simulink model "model"  (R2014a)
settings: Solver=VariableStepAuto  StartTime=0.0  StopTime=10.0  RelTol=1e-3
settings Model: Creator=GGX  LastModifiedBy=thinkpad
settings DataIOCC: LimitDataPoints=off  SaveFormat=Dataset
settings OptimizationCC: LifeSpan=auto  SimCompilerOptimization=off
settings DebuggingCC: MergeDetectMultiDrivingBlocksExec=error  SolverPrmCheckMsg=none  FcnCallInpInsideContextMsg=error  FrameProcessingCompatibilityMsg=error  SFUnexpectedBacktrackingDiag=error  SFNoUnconditionalDefaultTransitionDiag=error
settings HardwareCC: ProdBitPerPointer=64  ProdLargestAtomicFloat=Float  ProdIntDivRoundTo=Zero  ProdEndianess=LittleEndian  ProdWordSize=64  ProdHWDeviceType=Intel->x86-64 (Windows64)
settings ModelReferenceCC: PropagateSignalLabelsOutOfModel=on
settings RTWCC: RTWCompilerOptimization=off
settings GRTTargetCC: TargetLangStandard=C99 (ISO)  GeneratePreprocessorConditionals=Use local settings

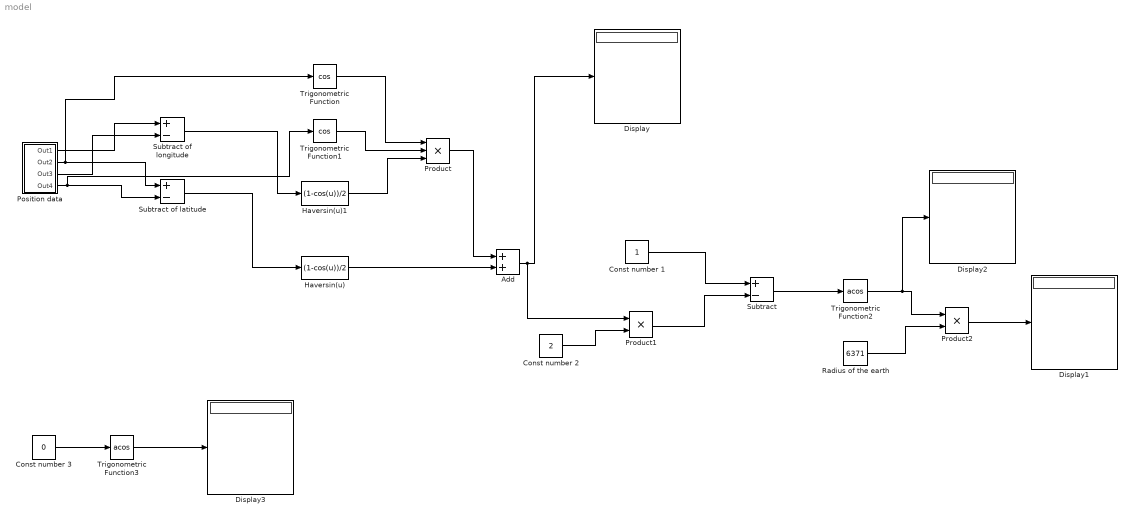
== system model ==
  Add : Sum
  Const number 1 : Constant  SampleTime=1
  Const number 2 : Constant  Value=2  SampleTime=1
  Const number 3 : Constant  Value=0  SampleTime=1
  Display{,1..3} (4 alike) : Display
  Haversin(u) : Fcn  Expr=(1-cos(u))/2
  Haversin(u)1 : Fcn  Expr=(1-cos(u))/2
  Position data : Subsystem
  Product : Product  Inputs=3
  Product1 : Product
  Product2 : Product
  Radius of the earth : Constant  Value=6371  SampleTime=1
  Subtract : Sum  Inputs=+-
  Subtract of latitude : Sum  Inputs=+-
  Subtract of longitude : Sum  Inputs=+-
  Trigonometric Function : Trigonometry  Operator=cos
  Trigonometric Function1 : Trigonometry  Operator=cos
  Trigonometric Function2 : Trigonometry  Operator=acos
  Trigonometric Function3 : Trigonometry  Operator=acos
  wires:
  Position data/2(Out2) -> Trigonometric Function/1, Subtract of latitude/1
  Position data/4(Out4) -> Trigonometric Function1/1, Subtract of latitude/2
  Position data/1(Out1) -> Subtract of longitude/1
  Position data/3(Out3) -> Subtract of longitude/2
  Subtract of latitude/1 -> Haversin(u)/1
  Haversin(u)/1 -> Add/2
  Subtract of longitude/1 -> Haversin(u)1/1
  Trigonometric Function/1 -> Product/1
  Trigonometric Function1/1 -> Product/2
  Haversin(u)1/1 -> Product/3
  Product/1 -> Add/1
  Add/1 -> Product1/1, Display/1
  Const number 1/1 -> Subtract/1
  Const number 2/1 -> Product1/2
  Product1/1 -> Subtract/2
  Subtract/1 -> Trigonometric Function2/1
  Trigonometric Function2/1 -> Display2/1, Product2/1
  Radius of the earth/1 -> Product2/2
  Product2/1 -> Display1/1
  Const number 3/1 -> Trigonometric Function3/1
  Trigonometric Function3/1 -> Display3/1

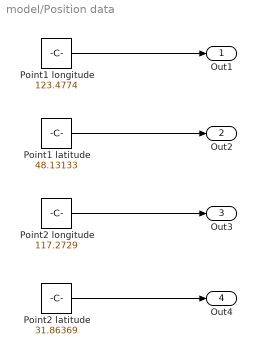
== system model/Position data ==
  Point1 latitude : Constant  Value=48.13133
  Point1 longitude : Constant  Value=123.4774
  Point2 latitude : Constant  Value=31.86369
  Point2 longitude : Constant  Value=117.2729
  Out1 : Outport
  Out2 : Outport  Port=2
  Out3 : Outport  Port=3
  Out4 : Outport  Port=4
  wires:
  Point2 longitude/1 -> Out3/1
  Point1 latitude/1 -> Out2/1
  Point1 longitude/1 -> Out1/1
  Point2 latitude/1 -> Out4/1
